simulink library "outp"  (R2021b)
settings: Solver=VariableStepAuto  StartTime=0.0  StopTime=10.0  RelTol=1e-3
undefined symbols (not defined in the file or in its folder): ENUM_PMMMODE_CHARGE, ENUM_PMMMODE_IDLE, ENUM_PMMMODE_INITIALIZE, ENUM_PMMMODE_POWERDOWN, ENUM_PMMMODE_SLEEP, slcm, TRUE
libraries: FVT_lib x736, hcu_lib x4, simulink x1
(part 1 of 8)
settings Model: Creator=13168  LastModifiedBy=yenst
settings SolverCC: AlgebraicLoopSolver=TrustRegion
settings DataIOCC: SaveFormat=Array  SignalLoggingSaveFormat=ModelDataLogs  ReturnWorkspaceOutputs=off
settings OptimizationCC: BlockReduction=off  BooleanDataType=off
settings DebuggingCC: SaveWithParameterizedLinksMsg=none  UnderspecifiedInitializationDetection=Classic  MergeDetectMultiDrivingBlocksExec=none  SignalResolutionControl=TryResolveAllWithWarning  SFMachineParentedDataDiag=warning
settings HardwareCC: TargetUnknown=on
settings ModelReferenceCC: PropagateSignalLabelsOutOfModel=off
settings ConfigComp: CovMetricSettings=dw  CovSaveCumulativeToWorkspaceVar=on  CovSaveSingleToWorkspaceVar=on

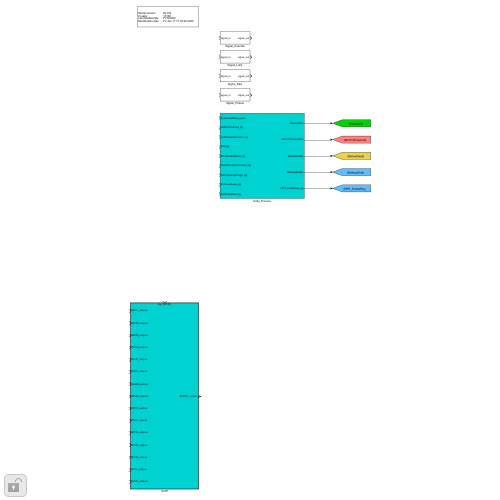
[thumbnail: Simulink's stored preview of the top-level diagram]
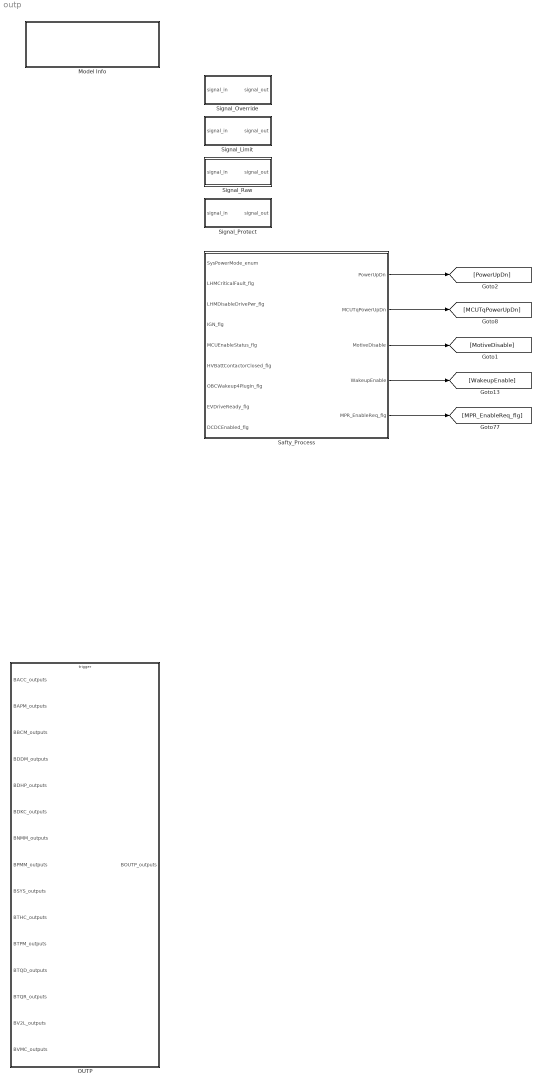
== system outp ==
  Model Info : Subsystem  LoadFcn=slcm LoadBlock;  InitFcn=slcm('UpdateAllCMBlocksInThisModelInit')  mask(CMBlock){InitialSaveTempField=, InitialBlockCM=None, BlockCM=None, Frame=on, SaveTempField=, DisplayStringWithTags=|, MaskDisplayString=Model Version        : 29.104\nCreator                   : 13168\nLast Modified By    : FVT22063\nModification date    : Fri Jan 17 17:30:42 2025, HorizontalTextAlignment=Left, LeftAlignmentValue=0.02, SourceBlockDiagram=outp, TagMaxNumber=20, CMTag1=, CMTag2=, CMTag3=, CMTag4=, CMTag5=, CMTag6=, CMTag7=, CMTag8=, CMTag9=, CMTag10=, CMTag11=, CMTag12=, CMTag13=, CMTag14=, CMTag15=, CMTag16=, CMTag17=, CMTag18=, CMTag19=, CMTag20=}
      mask DisplayStringWithTags=|
      | Model Version        : %<ModelVersion>\nCreator                   : %<Creator>\nLast Modified By    : %<LastModifiedBy>
      | Modification date    : %<LastModificationDate>
      mask help: This block allows revision control information to be displayed within the model.
      settings: CopyFcn=slcm CopyBlock;  DeleteFcn=slcm Cancel;  PostSaveFcn=slcm('UpdateAllCMBlocksInThisModel')  NameChangeFcn=slcm Rename;  OpenFcn=slcm
      mask Display: text(str2num(LeftAlignmentValue), 0.5, MaskDisplayString, 'HorizontalAlignment', HorizontalTextAlignment)
  OUTP : Subsystem
      settings: RTWSystemCode=Nonreusable function  RTWFcnNameOpts=Use subsystem name  RTWFileNameOpts=Use subsystem name
  Safty_Process : Subsystem
  Signal_Limit : Subsystem
  Signal_Override : Subsystem
  Signal_Protect : Subsystem
  Signal_Raw : Subsystem
  wires:
  Safty_Process/2(MCUTqPowerUpDn) -> [MCUTqPowerUpDn]
  Safty_Process/1(PowerUpDn) -> [PowerUpDn]
  Safty_Process/4(WakeupEnable) -> [WakeupEnable]
  Safty_Process/5(MPR_EnableReq_flg) -> [MPR_EnableReq_flg]
  Safty_Process/3(MotiveDisable) -> [MotiveDisable]

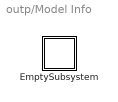
== system outp/Model Info ==
  EmptySubsystem : Subsystem
